simulink model "Problem_1"  (R2020b)
settings: Solver=VariableStepAuto  StartTime=0.0  StopTime=100  RelTol=1e-3
model workspace (MAT data in the model file):
  F = 1
  b = 50
  k = 100
  k1 = 4
  k12 = 25
  m1 = 100
  m2 = 0.25
libraries: simulink x1
settings Model: Creator=Saqlain  LastModifiedBy=mluser

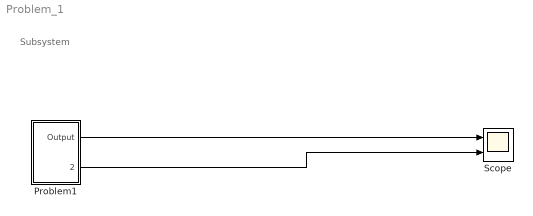
== system Problem_1 ==
  note: Subsystem
  Problem1 : Subsystem
  Scope : Scope  NumInputPorts=2
  wires:
  Problem1/1(Output) -> Scope/1
  Problem1/2(Output1) -> Scope/2

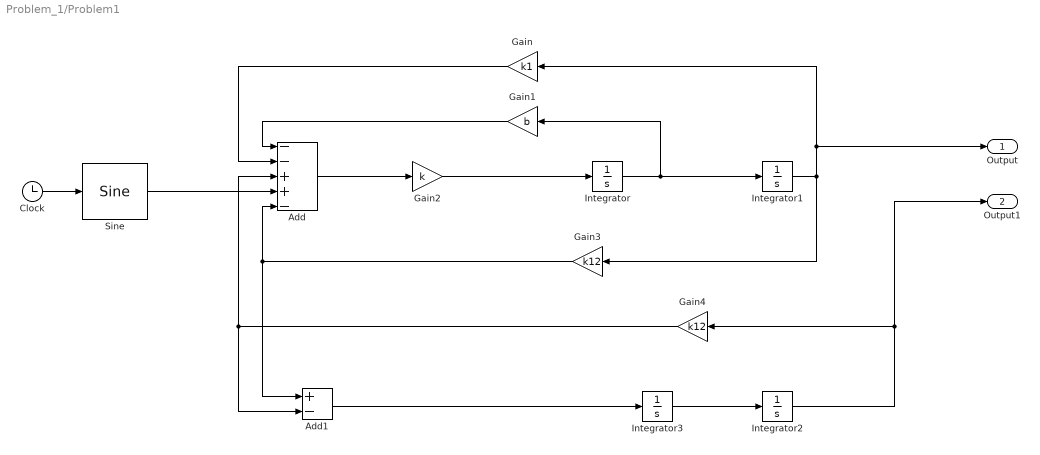
== system Problem_1/Problem1 ==
  Add : Sum  Inputs=--++-
  Add1 : Sum  Inputs=+-
  Clock : Clock
  Gain : Gain  Gain=k1
  Gain1 : Gain  Gain=b
  Gain2 : Gain  Gain=k
  Gain3 : Gain  Gain=k12
  Gain4 : Gain  Gain=k12
  Integrator{,1..3} (4 alike) : Integrator
  Sine : simulink/Lookup Tables/Sine  Formula=sin(2*pi*u)  NumDataPoints=(2^5)+1  OutputWordLength=16  InternalRulePriority=Speed
  Output : Outport
  Output1 : Outport  Port=2
  wires:
  Gain3/1 -> Add1/1, Add/5
  Gain/1 -> Add/2
  Gain4/1 -> Add1/2, Add/3
  Integrator/1 -> Gain1/1, Integrator1/1
  Clock/1 -> Sine/1
  Add/1 -> Gain2/1
  Integrator3/1 -> Integrator2/1
  Integrator1/1 -> Gain3/1, Output/1, Gain/1
  Integrator2/1 -> Output1/1, Gain4/1
  Gain1/1 -> Add/1
  Add1/1 -> Integrator3/1
  Sine/1 -> Add/4
  Gain2/1 -> Integrator/1
